simulink model "maglev"  (R2025b)
settings: Solver=VariableStepAuto  StartTime=0.0  StopTime=4  RelTol=1e-3
undefined symbols (not defined in the file): DiscIntNeverNeededParam, Kd, Ki, Kp, u0
settings Model: Creator=gusta  LastModifiedBy=gusta

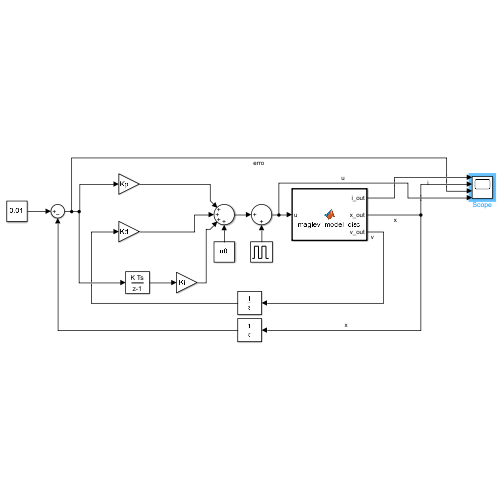
[thumbnail: Simulink's stored preview of the top-level diagram]
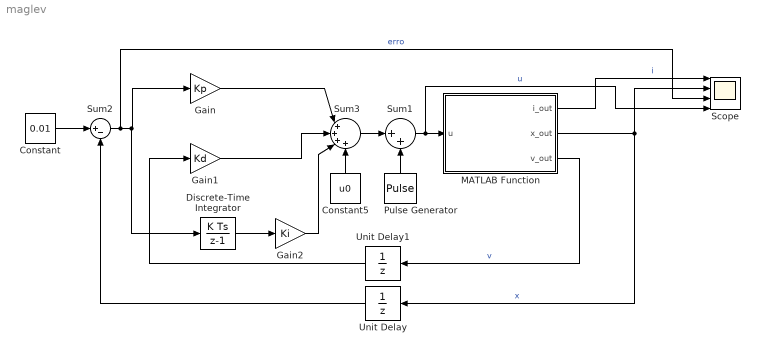
== system maglev ==
  Constant : Constant  Value=0.01
  Constant5 : Constant  Value=u0
  Discrete-Time Integrator : DiscreteIntegrator  SampleTime=0.001  ICPrevOutput=DiscIntNeverNeededParam  ICPrevScaledInput=DiscIntNeverNeededParam
  Gain : Gain  Gain=Kp
  Gain1 : Gain  Gain=Kd
  Gain2 : Gain  Gain=Ki
  MATLAB Function : MATLAB Function  TreatAsAtomicUnit=on
  Pulse Generator : DiscretePulseGenerator  PulseType=Time based  Amplitude=0  Period=10  PulseWidth=5
  Scope : Scope  NumInputPorts=4
      settings: ActiveDisplayYMinimum=-6.6629173109139392E+267  ActiveDisplayYMaximum=5.9966255798225472E+268
  Sum1 : Sum  Inputs=|++
  Sum2 : Sum  Inputs=|+-
  Sum3 : Sum  Inputs=|++++
  Unit Delay : UnitDelay  SampleTime=0.001  HasFrameUpgradeWarning=on
  Unit Delay1 : UnitDelay  SampleTime=0.001  HasFrameUpgradeWarning=on
  wires:
  MATLAB Function/2(x_out) -> Unit Delay/1, Scope/2  "x"
  MATLAB Function/1(i_out) -> Scope/1  "i"
  MATLAB Function/3(v_out) -> Unit Delay1/1  "v"
  Constant5/1 -> Sum3/4
  Constant/1 -> Sum2/1
  Sum2/1 -> Scope/3, Discrete-Time Integrator/1, Gain/1  "erro"
  Gain/1 -> Sum3/1
  Gain1/1 -> Sum3/2
  Sum3/1 -> Sum1/1
  Sum1/1 -> Scope/4, MATLAB Function/1(u)  "u"
  Pulse Generator/1 -> Sum1/2
  Discrete-Time Integrator/1 -> Gain2/1
  Gain2/1 -> Sum3/3
  Unit Delay/1 -> Sum2/2
  Unit Delay1/1 -> Gain1/1

== matlab function maglev/MATLAB Function ==
  data: u input; i_out output; x_out output; v_out output
function [i_out, x_out, v_out] = maglev_model_disc(u)

persistent i x v

% Parâmetros
m   = 0.022;
g   = 9.81;
kfm = 1.8632e-5;
kL  = 0.0000415;
Lb  = 0.4082238;
R   = 13.5;
Ts  = 0.001;

% Ponto de operação coerente para x0 = 1 cm
x0 = 0.01;
i0 = x0 * sqrt(m*g/kfm);

if isempty(i) 
    i = i0;
    x = x0;
    v = 0;
end

x_eff = max(x, 1e-4);

fm = kfm*(i^2)/(x_eff^2);
Bl = kfm*i/(x_eff^2);
L  = kL/x_eff + Lb;

di = (u - R*i - Bl*v)/L;
dx = v;
dv = g - fm/m;

i = i + Ts*di;
x = x + Ts*dx;
v = v + Ts*dv;

i_out = i;
x_out = x;
v_out = v;
end
